simulink model "ModelEnv_Test1"  (R2020b)
settings: Solver=VariableStepAuto  StartTime=0.0  StopTime=10  RelTol=1e-3
values from neighbouring files (symbols this model uses):
  Atz = -0.15    [AgentSaboteur.m]    (also in Test1_code.m; TesterUnAgent.m; test_RL_code.m; test_RL_code_v2.m)
  Bd = 0.03    [AgentSaboteur.m]    (also in Test1_code.m; TesterUnAgent.m; test_RL_code.m; test_RL_code_v2.m)
  Tz_init = Tout(1)    [AgentSaboteur.m]    (also in Test1_code.m; TesterUnAgent.m; testBlanc.m; test_RL_code.m)
libraries: dspsrcs4 x1
settings Model: Creator=masdoua1  LastModifiedBy=masdoua1
settings SolverCC: AlgebraicLoopSolver=LineSearch

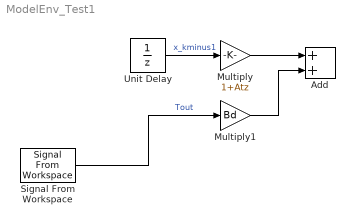
== system ModelEnv_Test1 ==
  Add : Sum
  Multiply : Gain  Gain=1+Atz
  Multiply1 : Gain  Gain=Bd
  Signal From Workspace : dspsrcs4/Signal From Workspace  X=Tout  Ts=1  nsamps=1  OutputAfterFinalValue=Setting to zero  ignoreOrWarnInputAndFrameLengths=off  OutputFrames=off
  Unit Delay : UnitDelay  InitialCondition=Tz_init  HasFrameUpgradeWarning=on
  wires:
  Unit Delay/1 -> Multiply/1  "x_kminus1"
  Multiply/1 -> Add/1
  Signal From Workspace/1 -> Multiply1/1  "Tout"
  Multiply1/1 -> Add/2
